simulink model "Buttons"  (R2019b)
settings: Solver=FixedStepAuto  StartTime=0.0  StopTime=Inf  RelTol=1e-3  SampleTimeConstraint=STIndependent
undefined symbols (not defined in the file): BIT_MASK_GREEN_BUTTON, BIT_MASK_MASTER_SWITCH, BIT_MASK_RED_BUTTON, BUTTONS_REGISTER, char2dec
libraries: simulink x5
Description:
  | % Copyright 2019 The MathWorks, Inc.
settings Model: DataDictionary=Parameters.sldd  EnableAccessToBaseWorkspace=off  EnablePacing=on  Creator=sdupertu  LastModifiedBy=sdupertu
settings DataIOCC: SaveOutput=off  SaveTime=off
settings OptimizationCC: DefaultParameterBehavior=Inlined  EnhancedBackFolding=on  PassReuseOutputArgsAs=Individual arguments  OptimizeBlockOrder=speed  DifferentSizesBufferReuse=on  OptimizationCustomize=off  EfficientTunableParamExpr=on
settings DebuggingCC: ParameterTunabilityLossMsg=error  PregeneratedLibrarySubsystemCodeDiagnostic=none  ArithmeticOperatorsInVariantConditions=warning
settings ModelReferenceCC: EnableParallelModelReferenceBuilds=on
settings SFSimCC: SimUseLocalCustomCode=off  MATLABDynamicMemAlloc=off  CustomCodeUndefinedFunction=UseInterfaceOnly
settings RTWCC: SystemTargetFile=ert.tlc  TemplateMakefile=ert_default_tmf  GenerateReport=on  RTWUseLocalCustomCode=off  IncludeHyperlinkInReport=on  LaunchReport=on  GenerateTraceInfo=on  GenerateTraceReport=on  GenerateTraceReportSl=on  GenerateTraceReportSf=on  GenerateTraceReportEml=on  GenerateWebview=on  GenerateCodeMetricsReport=on
settings CodeAppCC: ForceParamTrailComments=on  IgnoreCustomStorageClasses=off  MaxIdLength=61  OperatorAnnotations=on  SimulinkDataObjDesc=on  SFDataObjDesc=on  InsertBlockDesc=on
settings ERTTargetCC: TargetLangStandard=C99 (ISO)  GenerateSampleERTMain=on  InlinedParameterPlacement=NonHierarchical  ERTCustomFileTemplate=example_file_process.tlc

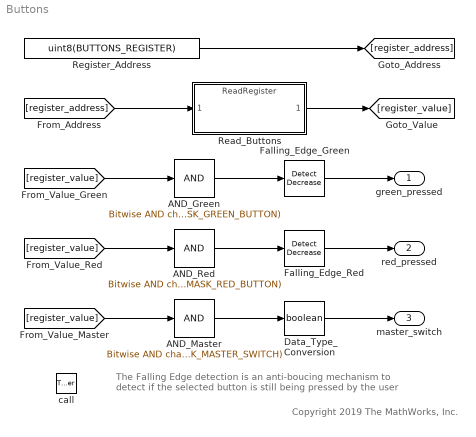
== system Buttons ==
  note: The Falling Edge detection is an anti-boucing mechanism to
      | detect if the selected button is still being pressed by the user
  note: Copyright 2019 The MathWorks, Inc.
  call : TriggerPort  TriggerType=function-call  VariantControl=Variant  PortDimensions=1  TriggerSignalSampleTime=[0.001,0]
  AND_Green : simulink/Logic and Bit Operations/Bitwise Operator  logicop=AND  UseBitMask=on  BitMask=char2dec(BIT_MASK_GREEN_BUTTON)  BitMaskRealWorld=Stored Integer
  AND_Master : simulink/Logic and Bit Operations/Bitwise Operator  logicop=AND  UseBitMask=on  BitMask=char2dec(BIT_MASK_MASTER_SWITCH)  BitMaskRealWorld=Stored Integer
  AND_Red : simulink/Logic and Bit Operations/Bitwise Operator  logicop=AND  UseBitMask=on  BitMask=char2dec(BIT_MASK_RED_BUTTON)  BitMaskRealWorld=Stored Integer
  Data_Type_Conversion : DataTypeConversion  OutDataTypeStr=boolean
  Falling_Edge_Green : simulink/Logic and Bit Operations/Detect Decrease  vinit=0  OutDataTypeStr=boolean
  Falling_Edge_Red : simulink/Logic and Bit Operations/Detect Decrease  vinit=0  OutDataTypeStr=boolean
  Read_Buttons : ModelReference  ModelNameDialog=ReadRegister.slx  SimulationMode=Normal  ModelReferenceVersion=1.122
  Register_Address : Constant  Value=uint8(BUTTONS_REGISTER)  SampleTime=-1
  green_pressed : Outport  OutDataTypeStr=boolean  PortDimensions=1  VectorParamsAs1DForOutWhenUnconnected=off
  red_pressed : Outport  Port=2  OutDataTypeStr=boolean  PortDimensions=1  VectorParamsAs1DForOutWhenUnconnected=off
  master_switch : Outport  Port=3  OutDataTypeStr=boolean  PortDimensions=1  VectorParamsAs1DForOutWhenUnconnected=off
  wires:
  Register_Address/1 -> [register_address]
  [register_address] -> Read_Buttons/1
  Read_Buttons/1 -> [register_value]
  [register_value] -> AND_Green/1
  AND_Green/1 -> Falling_Edge_Green/1
  Falling_Edge_Green/1 -> green_pressed/1
  AND_Red/1 -> Falling_Edge_Red/1
  Falling_Edge_Red/1 -> red_pressed/1
  [register_value] -> AND_Red/1
  AND_Master/1 -> Data_Type_Conversion/1
  [register_value] -> AND_Master/1
  Data_Type_Conversion/1 -> master_switch/1
